simulink model "SF5_1_1_stateflow_port_names"  (R2016b)
settings: Solver=FixedStepDiscrete  StartTime=0.0  StopTime=10.0  RelTol=1e-3  EnableMultiTasking=on
PostLoadFcn:
  | % -------------------------------------------------------------------
  | %  Generated by MATLAB on 7-Feb-2017 11:23:17
  | %  MATLAB version: 9.1.0.441655 (R2016b)
  | % -------------------------------------------------------------------
  | 
  | 
  | diffName = Simulink.Signal;
  | diffName.CoderInfo.StorageClass = 'ExportedGlobal';
  | diffName.CoderInfo.Alias = '';
  | diffName.CoderInfo.Alignment = -1;
  | diffName.Description = '';
  | diffName.DataType = 'auto';
  | diffName.Min = [];
  | diffName.Max = [];
  | diffName.DocUnits = '';
  | diffName.Dimensions = -1;
  | diffName.DimensionsMode = 'auto';
  | diffName.Complexity = 'auto';
  | diffName.SampleTime = -1;
  | diffName.InitialValue = '';
  | 
  | myinput = Simulink.Signal;
  | myinput.CoderInfo.StorageClass = 'ExportedGlobal';
  | myinput.CoderInfo.Alias = '';
  | myinput.CoderInfo.Alignment = -1;
  | myinput.Description = '';
  | myinput.DataType = 'auto';
  | myinput.Min = [];
  | myinput.Max = [];
  | myinput.DocUnits = '';
  | myinput.Dimensions = -1;
  | myinput.DimensionsMode = 'auto';
  | myinput.Complexity = 'auto';
  | myinput.SampleTime = -1;
  | myinput.InitialValue = '';
settings Model: Creator=amyyang  LastModifiedBy=amyyang
settings DataIOCC: LimitDataPoints=on
settings OptimizationCC: DefaultParameterBehavior=Inlined  LifeSpan=1
settings DebuggingCC: AllowSymbolicDim=off  SFUnusedDataAndEventsDiag=error  SFUnexpectedBacktrackingDiag=warning  SFNoUnconditionalDefaultTransitionDiag=warning  SFExecutionAtInitializationDiag=none
settings ModelReferenceCC: PropagateSignalLabelsOutOfModel=off
settings RTWCC: SystemTargetFile=ert.tlc  GenCodeOnly=on  TemplateMakefile=ert_default_tmf  Description=Embedded Coder  GenerateReport=on  IncludeHyperlinkInReport=on  LaunchReport=on  GenerateTraceInfo=on  GenerateTraceReport=on  GenerateTraceReportSl=on  GenerateTraceReportSf=on  GenerateTraceReportEml=on
settings CodeAppCC: IgnoreCustomStorageClasses=off
settings ERTTargetCC: GenerateSampleERTMain=on  InlinedParameterPlacement=NonHierarchical  ERTCustomFileTemplate=example_file_process.tlc  ConvertIfToSwitch=off  SuppressUnreachableDefaultCases=off
settings ConfigComp: CovMetricSettings=dw  CovHtmlReporting=on  CovSaveCumulativeToWorkspaceVar=on  CovSaveSingleToWorkspaceVar=on  CovExternalEMLEnable=off

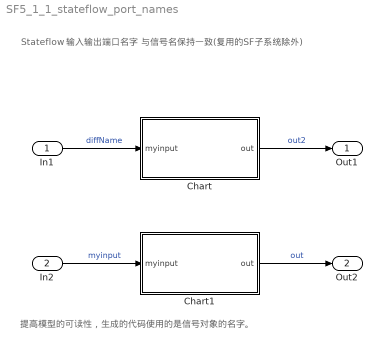
== system SF5_1_1_stateflow_port_names ==
  note: 提高模型的可读性，生成的代码使用的是信号对象的名字。
  note: Stateflow 输入输出端口名字
      | 与信号名保持一致(复用的SF子系统除外)
  In1 : Inport
  In2 : Inport  Port=2
  Chart : Stateflow chart  TreatAsAtomicUnit=on
  Chart1 : Stateflow chart  TreatAsAtomicUnit=on
  Out1 : Outport
  Out2 : Outport  Port=2
  wires:
  Chart/1(out) -> Out1/1  "out2"
  In1/1 -> Chart/1(myinput)  "diffName"
  Chart1/1(out) -> Out2/1  "out"
  In2/1 -> Chart1/1(myinput)  "myinput"

== stateflow chart SF5_1_1_stateflow_port_names/Chart1 ==
  (default) -> (junction 2) : {
      | out = param.*myinput;
      | }
  data: out output; myinput input; param parameter

== stateflow chart SF5_1_1_stateflow_port_names/Chart ==
  (default) -> (junction 2) : {
      | out = param.*myinput;
      | }
  data: out output; myinput input; param parameter double size=5
